simulink model "ThrusterCheckout"  (R2021a)
settings: Solver=FixedStepAuto  StartTime=0.0  StopTime=20  FixedStep=0.005  RelTol=1e-3  EnableMultiTasking=on
model workspace (MAT data in the model file):
  accelPhidget = [3707764736; 2; 1; 1; 1; 1]
  distPhidget1 = [3707764736; 2; 1; 1; 2; 2]
  distPhidget2 = [3707764736; 2; 1; 1; 3; 2]
  distPhidget3 = [3707764736; 2; 1; 1; 4; 2]
  distPhidget4 = [3707764736; 2; 1; 1; 5; 2]
  gyroPhidget = [3707764736; 2; 1; 1; 6; 3]
settings Model: EnablePacing=on  Creator=Andy  LastModifiedBy=Andy
settings SolverCC: AlgebraicLoopSolver=TrustRegion  PositivePriorityOrder=on
settings DataIOCC: SaveFormat=StructureWithTime  ReturnWorkspaceOutputs=off
settings OptimizationCC: EnhancedBackFolding=on  PassReuseOutputArgsAs=Individual arguments  ZeroExternalMemoryAtStartup=off  ZeroInternalMemoryAtStartup=off  MaxStackSize=64  OptimizeBlockOrder=speed  DifferentSizesBufferReuse=on  OptimizationCustomize=off  EfficientTunableParamExpr=on
settings DebuggingCC: ParameterTunabilityLossMsg=error  SFMachineParentedDataDiag=warning  ArithmeticOperatorsInVariantConditions=warning
settings HardwareCC: ProdBitPerPointer=32  ProdBitPerSizeT=32  ProdBitPerPtrDiffT=32  ProdLargestAtomicInteger=Long  ProdLargestAtomicFloat=Double  ProdWordSize=32  ProdHWDeviceType=ARM Compatible->ARM Cortex
settings ModelReferenceCC: ModelReferenceNumInstancesAllowed=Single
settings SFSimCC: MATLABDynamicMemAlloc=off  CustomCodeUndefinedFunction=UseInterfaceOnly  SimTargetLang=C++
settings RTWCC: SystemTargetFile=ert.tlc  HardwareBoard=Raspberry Pi  TLCOptions="-aInlineSetEventsForThisBaseRateFcn=TLC_TRUE -aSuppressMultiTaskScheduler=TLC_FALSE  -aRateBasedStepFcn=0"  GenCodeOnly=on  TemplateMakefile=ert_default_tmf  GenerateReport=on  Toolchain=GNU GCC Embedded Linux  BuildConfiguration=Faster Runs  IncludeHyperlinkInReport=on  LaunchReport=on  TargetLang=C++  GenerateTraceInfo=on  GenerateTraceReport=on  GenerateTraceReportSl=on  GenerateTraceReportSf=on  GenerateTraceReportEml=on
settings CodeAppCC: ForceParamTrailComments=on  IgnoreCustomStorageClasses=off  OperatorAnnotations=on  SimulinkDataObjDesc=on  SFDataObjDesc=on  InsertBlockDesc=on
settings ERTTargetCC: TargetLangStandard=C++03 (ISO)  MatFileLogging=on  CodeInterfacePackaging=C++ class  SupportVariableSizeSignals=on  MultiInstanceErrorCode=Warning  RootIOFormat=Structure reference

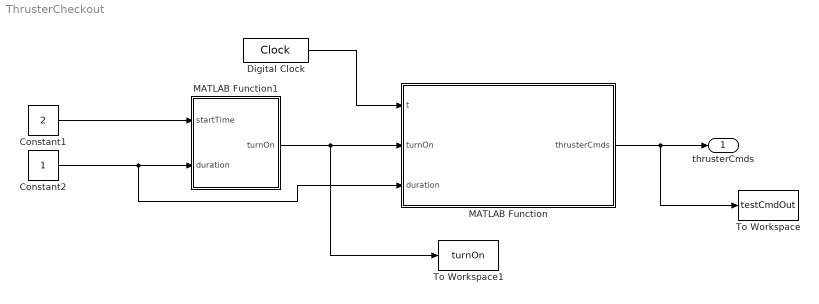
== system ThrusterCheckout ==
  Constant1 : Constant  Value=2
  Constant2 : Constant
  Digital Clock : DigitalClock  SampleTime=0.005
  MATLAB Function : MATLAB Function  TreatAsAtomicUnit=on
  MATLAB Function1 : MATLAB Function  TreatAsAtomicUnit=on
  To Workspace : ToWorkspace  VariableName=testCmdOut  SaveFormat=Timeseries  SampleTime=-1
  To Workspace1 : ToWorkspace  VariableName=turnOn  SaveFormat=Timeseries  SampleTime=-1
  thrusterCmds : Outport  VectorParamsAs1DForOutWhenUnconnected=off
  wires:
  MATLAB Function/1(thrusterCmds) -> To Workspace/1, thrusterCmds/1
  Digital Clock/1 -> MATLAB Function/1(t)
  Constant1/1 -> MATLAB Function1/1(startTime)
  Constant2/1 -> MATLAB Function/3(duration), MATLAB Function1/2(duration)
  MATLAB Function1/1(turnOn) -> To Workspace1/1, MATLAB Function/2(turnOn)

== matlab function ThrusterCheckout/MATLAB Function ==
  data: t input; thrusterCmds output; turnOn input; duration input
function thrusterCmds = fcn(t,turnOn,duration)
%   Thruster Layout
%     3       2   
%    4         1
%
%
%    5         8       
%     6       7          ^
%                        | 
%  + X -->             + Y 


% Default to zero each pass
thrusterCmds = zeros(8,1);

for i = 1:8
    if t >= turnOn(i) && t < turnOn(i) + duration
        thrusterCmds(i) = 1;
    end
end

== matlab function ThrusterCheckout/MATLAB Function1 ==
  data: turnOn output; startTime input; duration input
function turnOn = fcn(startTime,duration)

turnOn = zeros(8,1);

turnOn(1) = startTime;
for i = 2:8
    turnOn(i) = turnOn(i-1) + 2*duration;
end
